simulink model "QPSK"  (Simulink 6.3)
settings: Solver=ode45  StartTime=0.0  StopTime=30  RelTol=1e-3
libraries: xbsIndex_r4 x25, commrandsrc2 x1
settings Model: LastModifiedBy=Administrador
settings DebuggingCC: SolverPrmCheckMsg=none

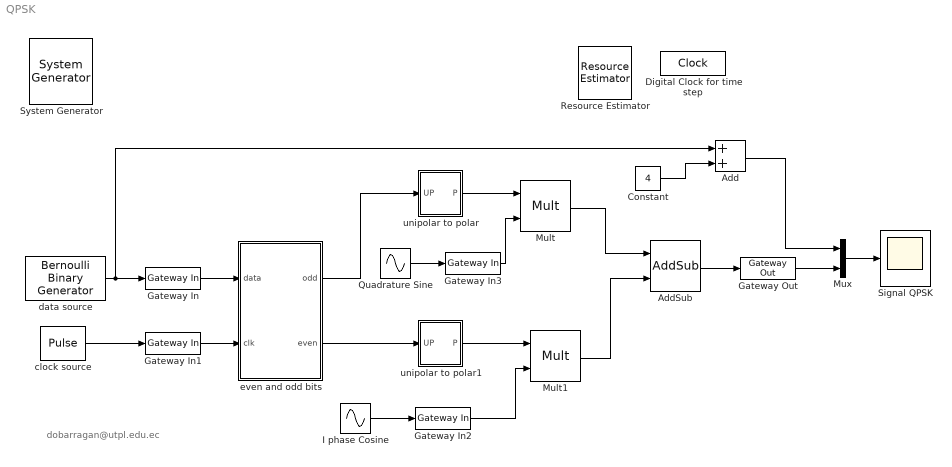
== system QPSK ==
  note: dobarragan@utpl.edu.ec
  " System Generator" : xbsIndex_r4/ System Generator  Tag=genX  xilinxfamily=Spartan3  part=xc3s200  speed=-4  package=ft256  synthesis_tool=XST  directory=./netlist  testbench=off  simulink_period=1/200  sysclk_period=10  incr_netlist=off  trim_vbits=Everywhere in SubSystem  dbl_ovrd=According to Block Masks  core_generation=According to Block Masks  run_coregen=off  deprecated_control=off  eval_field=0  block_type=sysgen
  Add : Sum  OutScaling=2^-10
  AddSub : xbsIndex_r4/AddSub  mode=Addition  use_carryin=off  use_carryout=off  en=off  latency=0  precision=User Defined  arith_type="Signed  (2's comp)"  n_bits=6  bin_pt=3  quantization="Round  (unbiased: +/- Inf)"  overflow=Saturate  dbl_ovrd=off  use_behavioral_HDL=off  pipelined=off  use_rpm=on  block_type=addsub
      settings: xl_area=[18 0 0 34 0 0 0]  block_version=VER_STRING_GOES_HERE
  Constant : Constant  Value=4
  Digital Clock for time step : DigitalClock  SampleTime=0.00001
  Gateway In : xbsIndex_r4/Gateway In  arith_type=Boolean  n_bits=1  bin_pt=0  quantization="Round  (unbiased: +/- Inf)"  overflow=Saturate  period=1/200  dbl_ovrd=off  timing_constraint=None  locs_specified=off  LOCs={}  block_type=gatewayin
      settings: infoedit="Gateway in block.  Converts inputs of type Simulink integer, double and fixed point to  Xilinx fixed point type.<P><P>Hardware notes:  In hardware these blocks become top level input ports."  xl_area=[0 0 0 0 1 0 0]  block_version=VER_STRING_GOES_HERE
  Gateway In1 : xbsIndex_r4/Gateway In  arith_type=Boolean  n_bits=1  bin_pt=0  quantization="Round  (unbiased: +/- Inf)"  overflow=Saturate  period=1/200  dbl_ovrd=off  timing_constraint=None  locs_specified=off  LOCs={}  block_type=gatewayin
      settings: infoedit="Gateway in block.  Converts inputs of type Simulink integer, double and fixed point to  Xilinx fixed point type.<P><P>Hardware notes:  In hardware these blocks become top level input ports."  xl_area=[0 0 0 0 1 0 0]  block_version=VER_STRING_GOES_HERE
  Gateway In2 : xbsIndex_r4/Gateway In  arith_type="Signed  (2's comp)"  n_bits=6  bin_pt=4  quantization="Round  (unbiased: +/- Inf)"  overflow=Saturate  period=1/200  dbl_ovrd=off  timing_constraint=None  locs_specified=off  LOCs={}  block_type=gatewayin
      settings: infoedit="Gateway in block.  Converts inputs of type Simulink integer, double and fixed point to  Xilinx fixed point type.<P><P>Hardware notes:  In hardware these blocks become top level input ports."  xl_area=[0 0 0 0 6 0 0]  block_version=VER_STRING_GOES_HERE
  Gateway In3 : xbsIndex_r4/Gateway In  arith_type="Signed  (2's comp)"  n_bits=6  bin_pt=4  quantization="Round  (unbiased: +/- Inf)"  overflow=Saturate  period=1/200  dbl_ovrd=off  timing_constraint=None  locs_specified=off  LOCs={}  block_type=gatewayin
      settings: infoedit="Gateway in block.  Converts inputs of type Simulink integer, double and fixed point to  Xilinx fixed point type.<P><P>Hardware notes:  In hardware these blocks become top level input ports."  xl_area=[0 0 0 0 6 0 0]  block_version=VER_STRING_GOES_HERE
  Gateway Out : xbsIndex_r4/Gateway Out  hdl_port=on  timing_constraint=None  locs_specified=off  LOCs={}  block_type=gatewayout
      settings: infoedit="Gateway out block.  Converts Xilinx fixed point inputs into ouputs of type Simulink integer, double, or fixed point.<P><P>Hardware notes:  In hardware these blocks become top level output ports or are discarded, depending on how they are configured."  xl_area=[0 0 0 0 6 0 0]  block_version=VER_STRING_GOES_HERE
  I phase Cosine : Sin  SineType=Sample based  Samples=100  SampleTime=1/200  Offset=25
  Mult : xbsIndex_r4/Mult  precision=Full  arith_type="Signed  (2's comp)"  n_bits=16  bin_pt=14  quantization=Truncate  overflow=Wrap  en=off  latency=3  dbl_ovrd=off  use_behavioral_HDL=off  use_embedded=off  pipeline=on  use_rpm=on  placement_style=Rectangular shape  block_type=mult
      settings: infoedit=Hardware notes: To use the internal pipeline stage of the dedicated multiplier you must select 'Pipeline for maximum performance'.  xl_area=[18 33 0 23 0 0 0]  block_version=VER_STRING_GOES_HERE
  Mult1 : xbsIndex_r4/Mult  precision=Full  arith_type="Signed  (2's comp)"  n_bits=16  bin_pt=14  quantization=Truncate  overflow=Wrap  en=off  latency=3  dbl_ovrd=off  use_behavioral_HDL=off  use_embedded=off  pipeline=on  use_rpm=on  placement_style=Rectangular shape  block_type=mult
      settings: infoedit=Hardware notes: To use the internal pipeline stage of the dedicated multiplier you must select 'Pipeline for maximum performance'.  xl_area=[18 33 0 23 0 0 0]  block_version=VER_STRING_GOES_HERE
  Mux : Mux  Inputs=2
  Quadrature Sine : Sin  SineType=Sample based  Samples=100  SampleTime=1/200  Offset=50
  Resource Estimator : xbsIndex_r4/Resource Estimator  Tag=resEstTag  Slices=103  FFs=77  BRAMs=0  LUTs=176  IOBs=0  EBMs=0  TBUFs=0  xl_use_estimator_area=off  est_options=Post Map  block_type=resource_estimator
      settings: AttributesFormatString=Resource\nEstimator
  Signal QPSK : Scope
      settings: TimeRange=10  YMin=-8  YMax=8  SaveName=ScopeData2
  clock source : DiscretePulseGenerator  Period=200  PulseWidth=100  SampleTime=1/200
  data source : commrandsrc2/Bernoulli Binary Generator  P=0.5  seed=61  Ts=.5  frameBased=off  sampPerFrame=1  orient=off  outDataType=double
  even and odd bits : Subsystem
  unipolar to polar : Subsystem
  unipolar to polar1 : Subsystem
  wires:
  data source/1 -> Gateway In/1, Add/1
  clock source/1 -> Gateway In1/1
  Gateway In/1 -> even and odd bits/1(data)
  Gateway In1/1 -> even and odd bits/2(clk)
  even and odd bits/1(odd) -> unipolar to polar/1(UP)
  even and odd bits/2(even) -> unipolar to polar1/1(UP)
  unipolar to polar/1(P) -> Mult/1
  unipolar to polar1/1(P) -> Mult1/1
  Mult/1 -> AddSub/1
  Mult1/1 -> AddSub/2
  Quadrature Sine/1 -> Gateway In3/1
  I phase Cosine/1 -> Gateway In2/1
  Gateway In3/1 -> Mult/2
  Gateway In2/1 -> Mult1/2
  AddSub/1 -> Gateway Out/1
  Mux/1 -> Signal QPSK/1
  Gateway Out/1 -> Mux/2
  Constant/1 -> Add/2
  Add/1 -> Mux/1

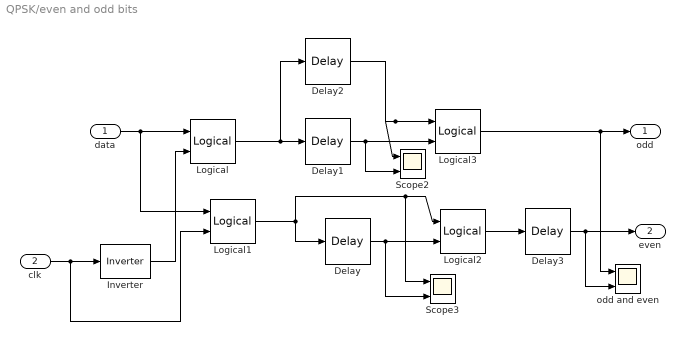
== system QPSK/even and odd bits ==
  data : Inport
  clk : Inport  Port=2
  Delay : xbsIndex_r4/Delay  en=off  latency=100  dbl_ovrd=off  reg_retiming=off  block_type=delay
      settings: infoedit=Hardware notes: A delay line is a chain, each link of which is an SRL16 followed by a flip-flop. If register retiming is enabled, the delay line is a chain of flip-flops.  xl_area=[6 6 0 6 0 0 0]  block_version=VER_STRING_GOES_HERE
  Delay1 : xbsIndex_r4/Delay  en=off  latency=200  dbl_ovrd=off  reg_retiming=off  block_type=delay
      settings: infoedit=Hardware notes: A delay line is a chain, each link of which is an SRL16 followed by a flip-flop. If register retiming is enabled, the delay line is a chain of flip-flops.  xl_area=[12 12 0 12 0 0 0]  block_version=VER_STRING_GOES_HERE
  Delay2 : xbsIndex_r4/Delay  en=off  latency=100  dbl_ovrd=off  reg_retiming=off  block_type=delay
      settings: infoedit=Hardware notes: A delay line is a chain, each link of which is an SRL16 followed by a flip-flop. If register retiming is enabled, the delay line is a chain of flip-flops.  xl_area=[6 6 0 6 0 0 0]  block_version=VER_STRING_GOES_HERE
  Delay3 : xbsIndex_r4/Delay  en=off  latency=200  dbl_ovrd=off  reg_retiming=off  block_type=delay
      settings: infoedit=Hardware notes: A delay line is a chain, each link of which is an SRL16 followed by a flip-flop. If register retiming is enabled, the delay line is a chain of flip-flops.  xl_area=[36 72 0 72 0 0 0]  block_version=VER_STRING_GOES_HERE
  Inverter : xbsIndex_r4/Inverter  en=off  latency=0  dbl_ovrd=off  block_type=inv
      settings: xl_area=[0 0 0 0 0 0 0]  block_version=VER_STRING_GOES_HERE
  Logical : xbsIndex_r4/Logical  logical_function=AND  inputs=2  en=off  latency=0  precision=Full  arith_type=Unsigned  n_bits=16  bin_pt=0  align_bp=on  dbl_ovrd=off  block_type=logical
      settings: xl_area=[1 0 0 1 0 0 0]  block_version=VER_STRING_GOES_HERE
  Logical1 : xbsIndex_r4/Logical  logical_function=AND  inputs=2  en=off  latency=0  precision=Full  arith_type=Unsigned  n_bits=16  bin_pt=0  align_bp=on  dbl_ovrd=off  block_type=logical
      settings: xl_area=[1 0 0 1 0 0 0]  block_version=VER_STRING_GOES_HERE
  Logical2 : xbsIndex_r4/Logical  logical_function=XOR  inputs=2  en=off  latency=2  precision=User Defined  arith_type=Unsigned  n_bits=6  bin_pt=3  align_bp=on  dbl_ovrd=off  block_type=logical
      settings: xl_area=[4 7 0 1 0 0 0]  block_version=VER_STRING_GOES_HERE
  Logical3 : xbsIndex_r4/Logical  logical_function=XOR  inputs=2  en=off  latency=1  precision=User Defined  arith_type=Unsigned  n_bits=2  bin_pt=0  align_bp=on  dbl_ovrd=off  block_type=logical
      settings: xl_area=[1 1 0 1 0 0 0]  block_version=VER_STRING_GOES_HERE
  Scope2 : Scope  NumInputPorts=2
      settings: YMin=-2~-2  YMax=2~2  SaveName=ScopeData6
  Scope3 : Scope  NumInputPorts=2
      settings: YMin=-2~-2  YMax=2~2
  odd and even : Scope  NumInputPorts=2
      settings: YMin=-2~-2  YMax=2~2  SaveName=ScopeData4
  odd : Outport
  even : Outport  Port=2
  wires:
  clk/1 -> Logical1/2, Inverter/1
  Inverter/1 -> Logical/2
  Logical1/1 -> Delay/1, Logical2/1, Scope3/1
  Delay/1 -> Logical2/2, Scope3/2
  Logical/1 -> Delay1/1, Delay2/1
  Delay1/1 -> Logical3/2, Scope2/2
  Logical3/1 -> odd/1, odd and even/1
  data/1 -> Logical/1, Logical1/1
  Delay2/1 -> Logical3/1, Scope2/1
  Logical2/1 -> Delay3/1
  Delay3/1 -> even/1, odd and even/2

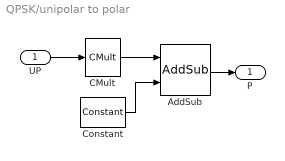
== system QPSK/unipolar to polar ==
  UP : Inport
  AddSub : xbsIndex_r4/AddSub  mode=Subtraction  use_carryin=off  use_carryout=off  en=off  latency=0  precision=User Defined  arith_type="Signed  (2's comp)"  n_bits=3  bin_pt=0  quantization=Truncate  overflow=Wrap  dbl_ovrd=off  use_behavioral_HDL=off  pipelined=off  use_rpm=on  block_type=addsub
      settings: xl_area=[2 0 0 3 0 0 0]  block_version=VER_STRING_GOES_HERE
  CMult : xbsIndex_r4/CMult  const=2  const_n_bits=2  const_bin_pt=0  en=off  latency=0  precision=Full  arith_type="Signed  (2's comp)"  n_bits=16  bin_pt=14  quantization=Truncate  overflow=Wrap  dbl_ovrd=off  use_behavioral_HDL=off  mem_type=Distributed RAM  placement_style=Rectangular Shape  pipeline=off  use_rpm=off  block_type=cmult
      settings: xl_area=[0 0 0 0 0 0 0]  block_version=VER_STRING_GOES_HERE
  Constant : xbsIndex_r4/Constant  arith_type=Unsigned  const=1  n_bits=1  bin_pt=0  explicit_period=off  period=1  equ=P=C  opselect=C  inp2=PCIN>>17  opr=+  inp1=P  carry=CIN  dbl_ovrd=off  block_type=constant
      settings: block_version=VER_STRING_GOES_HERE
  P : Outport
  wires:
  CMult/1 -> AddSub/1
  Constant/1 -> AddSub/2
  UP/1 -> CMult/1
  AddSub/1 -> P/1

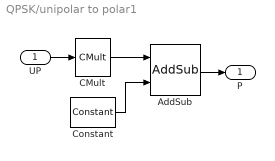
== system QPSK/unipolar to polar1 ==
  UP : Inport
  AddSub : xbsIndex_r4/AddSub  mode=Subtraction  use_carryin=off  use_carryout=off  en=off  latency=0  precision=User Defined  arith_type="Signed  (2's comp)"  n_bits=3  bin_pt=0  quantization=Truncate  overflow=Wrap  dbl_ovrd=off  use_behavioral_HDL=off  pipelined=off  use_rpm=on  block_type=addsub
      settings: xl_area=[2 0 0 3 0 0 0]  block_version=VER_STRING_GOES_HERE
  CMult : xbsIndex_r4/CMult  const=2  const_n_bits=2  const_bin_pt=0  en=off  latency=0  precision=Full  arith_type="Signed  (2's comp)"  n_bits=16  bin_pt=14  quantization=Truncate  overflow=Wrap  dbl_ovrd=off  use_behavioral_HDL=off  mem_type=Distributed RAM  placement_style=Rectangular Shape  pipeline=off  use_rpm=off  block_type=cmult
      settings: xl_area=[0 0 0 0 0 0 0]  block_version=VER_STRING_GOES_HERE
  Constant : xbsIndex_r4/Constant  arith_type=Unsigned  const=1  n_bits=1  bin_pt=0  explicit_period=off  period=1  equ=P=C  opselect=C  inp2=PCIN>>17  opr=+  inp1=P  carry=CIN  dbl_ovrd=off  block_type=constant
      settings: block_version=VER_STRING_GOES_HERE
  P : Outport
  wires:
  AddSub/1 -> P/1
  UP/1 -> CMult/1
  Constant/1 -> AddSub/2
  CMult/1 -> AddSub/1
